simulink model "Circuito_RC"  (R2019a)
settings: Solver=VariableStepAuto  StartTime=0.0  StopTime=10  RelTol=1e-3
values from neighbouring files (symbols this model uses):
  C = input('Capacitância: ')    [CircuitoRC_run.m]
  R = input('Resistência: ')    [CircuitoRC_run.m]
  Vo = input('Tensão incial: ')    [CircuitoRC_run.m]
settings Model: Creator=mateu  LastModifiedBy=mateu

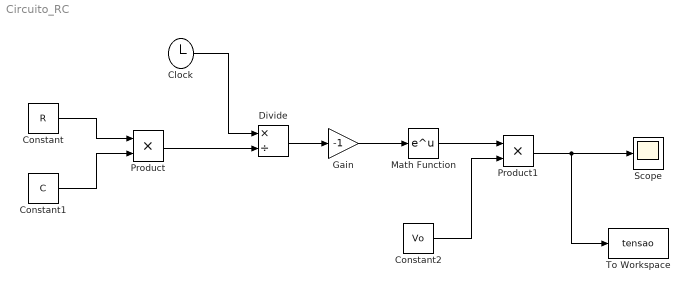
== system Circuito_RC ==
  Clock : Clock
  Constant : Constant  Value=R
  Constant1 : Constant  Value=C
  Constant2 : Constant  Value=Vo
  Divide : Product  Inputs=*/
  Gain : Gain  Gain=-1
  Math Function : Math  SaturateOnIntegerOverflow=on
  Product : Product
  Product1 : Product
  Scope : Scope
  To Workspace : ToWorkspace  VariableName=tensao  SaveFormat=Timeseries  SampleTime=-1
  wires:
  Constant/1 -> Product/1
  Constant1/1 -> Product/2
  Product/1 -> Divide/2
  Clock/1 -> Divide/1
  Divide/1 -> Gain/1
  Gain/1 -> Math Function/1
  Math Function/1 -> Product1/1
  Constant2/1 -> Product1/2
  Product1/1 -> To Workspace/1, Scope/1
